simulink model "Transmitter"  (R2015a)
settings: Solver=ode45  StartTime=0.0  StopTime=10.0  RelTol=1e-3
libraries: xpcutilitieslib x1, xpciplib x1, xpcrtudplib x1
settings Model: xpc_rtwmakecfg_data=_xpcetherlib__xpcether8255xlib__xpcetherGbElib_  Creator=Dominik  LastModifiedBy=Dominik

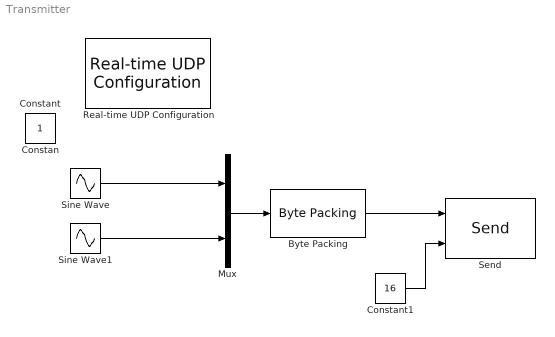
== system Transmitter ==
  "Byte Packing " : xpcutilitieslib/Byte Packing   MaskPackedDataType=uint8  MaskUnpackedDataTypes={'double'}  MaskAlignment=1
  Constant1 : Constant  Value=16
  Mux : Mux  Inputs=2
  "Real-time UDP Configuration " : xpciplib/Real-time UDP  Configuration   ID=1  IpAddress=30.30.30.1  SubnetMask=255.255.255.0  Gateway=0.0.0.0  EthDrv=Intel Gigabit  PciBus=5  PciSlot=0  udpID=0
  "Send " : xpcrtudplib/Send   ID=1  Send1=30.30.30.2  Send2=25000  Send3=-1  Send4=-1  udpID=0
  Sine Wave : Sin  SampleTime=0
  Sine Wave1 : Sin  SampleTime=0
  Constan : Constant  IOType=siggen
  Constant : Constant  IOType=siggen
  wires:
  Sine Wave1/1 -> Mux/2
  Sine Wave/1 -> Mux/1
  Mux/1 -> "Byte Packing "/1
  "Byte Packing "/1 -> "Send "/1
  Constant1/1 -> "Send "/2
